simulink model "lb52"  (R2020b)
settings: Solver=VariableStepAuto  StartTime=0.0  StopTime=4  MaxStep=0.01  RelTol=1e-3
libraries: simulink_extras x2
settings Model: Creator=nda020101  LastModifiedBy=nda020101

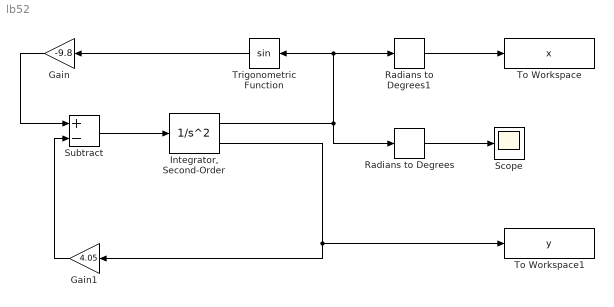
== system lb52 ==
  Gain : Gain  Gain=-9.8
  Gain1 : Gain  Gain=4.05
  "Integrator, Second-Order" : SecondOrderIntegrator  ICX=-pi+0.0015  ICDXDT=1
  Radians to Degrees : simulink_extras/Transformations/Radians to Degrees
  Radians to Degrees1 : simulink_extras/Transformations/Radians to Degrees
  Scope : Scope
  Subtract : Sum  Inputs=+-
  To Workspace : ToWorkspace  VariableName=x  SaveFormat=Timeseries  SampleTime=-1
  To Workspace1 : ToWorkspace  VariableName=y  SaveFormat=Timeseries  SampleTime=-1
  Trigonometric Function : Trigonometry
  wires:
  Radians to Degrees/1 -> Scope/1
  Radians to Degrees1/1 -> To Workspace/1
  Subtract/1 -> "Integrator, Second-Order"/1
  Gain1/1 -> Subtract/2
  Gain/1 -> Subtract/1
  Trigonometric Function/1 -> Gain/1
  "Integrator, Second-Order"/2 -> Gain1/1, To Workspace1/1
  "Integrator, Second-Order"/1 -> Radians to Degrees/1, Radians to Degrees1/1, Trigonometric Function/1
